simulink model "erg"  (R2021b)
settings: Solver=VariableStepAuto  StartTime=0.0  StopTime=TT  RelTol=1e-3
values from neighbouring files (symbols this model uses):
  A = [0,0,1,0 ... (first row only)    [erg_first_steps.m]
  B = [0,0 ... (first row only)    [erg_first_steps.m]
  constr = [10;10;0;0;0;0;0;0]    [erg_first_steps.m]
  delta = 1    [erg_first_steps.m]    (also in erg_point_testing.m = -1)
  Kd = 2*zeta*wn    [erg_first_steps.m]    (also in symplectic_euler.m = 2.556)
  Kp = umax/max(r)    [erg_first_steps.m]    (also in symplectic_euler.m = 3.3333)
  r = [11;9.9]    [erg_first_steps.m]    (also in erg_point_testing.m = [7;11])
  Ts = 0.1    [erg_first_steps.m]
  x0 = zeros(4,1)    [erg_first_steps.m]    (also in symplectic_euler.m = [0;0])
  zeta = 2    [erg_first_steps.m]    (also in erg_point_testing.m)
settings Model: Creator=jon-h  LastModifiedBy=jon-h

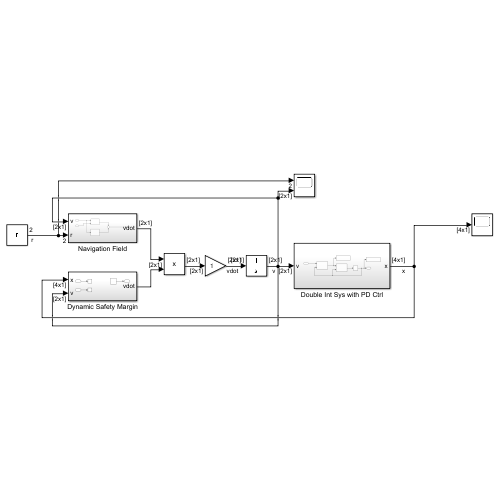
[thumbnail: Simulink's stored preview of the top-level diagram]
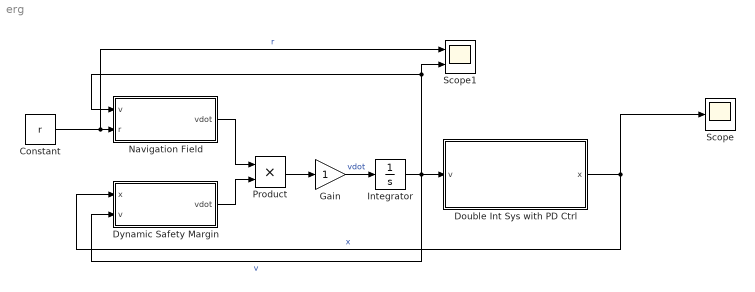
== system erg ==
  Constant : Constant  Value=r  SampleTime=Ts
  Double Int Sys with PD Ctrl : Subsystem
  Dynamic Safety Margin : Subsystem
  Gain : Gain
  Integrator : Integrator  InitialCondition=r
  Navigation Field : Subsystem
  Product : Product
  Scope : Scope
  Scope1 : Scope  NumInputPorts=2
  wires:
  Double Int Sys with PD Ctrl/1(x) -> Dynamic Safety Margin/1(x), Scope/1  "x"
  Integrator/1 -> Dynamic Safety Margin/2(v), Scope1/2, Navigation Field/1(v), Double Int Sys with PD Ctrl/1(v)  "v"
  Constant/1 -> Scope1/1, Navigation Field/2(r)  "r"
  Navigation Field/1(vdot) -> Product/1
  Dynamic Safety Margin/1(vdot) -> Product/2
  Gain/1 -> Integrator/1  "vdot"
  Product/1 -> Gain/1

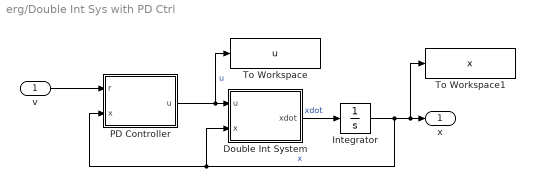
== system erg/Double Int Sys with PD Ctrl ==
  v : Inport
  Double Int System : MATLAB Function  TreatAsAtomicUnit=on
  Integrator : Integrator  InitialCondition=x0
  PD Controller : MATLAB Function  TreatAsAtomicUnit=on
  To Workspace : ToWorkspace  VariableName=u  SaveFormat=Timeseries  SampleTime=-1
  To Workspace1 : ToWorkspace  VariableName=x  SaveFormat=Timeseries  SampleTime=-1
  x : Outport
  wires:
  Integrator/1 -> To Workspace1/1, x/1, Double Int System/2(x), PD Controller/2(x)  "x"
  PD Controller/1(u) -> To Workspace/1, Double Int System/1(u)  "u"
  Double Int System/1(xdot) -> Integrator/1  "xdot"
  v/1 -> PD Controller/1(r)

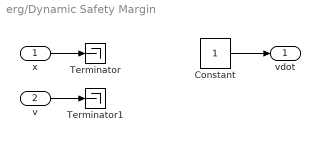
== system erg/Dynamic Safety Margin ==
  x : Inport
  v : Inport  Port=2
  Constant : Constant
  Terminator : Terminator
  Terminator1 : Terminator
  vdot : Outport
  wires:
  Constant/1 -> vdot/1
  x/1 -> Terminator/1
  v/1 -> Terminator1/1

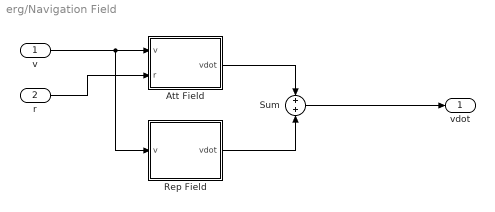
== system erg/Navigation Field ==
  v : Inport
  r : Inport  Port=2
  Att Field : MATLAB Function  TreatAsAtomicUnit=on
  Rep Field : MATLAB Function  TreatAsAtomicUnit=on
  Sum : Sum  Inputs=+|+
  vdot : Outport
  wires:
  v/1 -> Att Field/1(v), Rep Field/1(v)
  r/1 -> Att Field/2(r)
  Att Field/1(vdot) -> Sum/1
  Rep Field/1(vdot) -> Sum/2
  Sum/1 -> vdot/1

== matlab function erg/Double Int Sys with PD Ctrl/PD Controller ==
  data: r input; u output; x input; Kp parameter; Kd parameter
function u = fcn(r,x,Kp,Kd)

u = [ - Kp*(x(1)-r(1)) - Kd*x(3) ;
      - Kp*(x(2)-r(2)) - Kd*x(4) ];

== matlab function erg/Double Int Sys with PD Ctrl/Double Int System ==
  data: u input; xdot output; x input; A parameter; B parameter
function xdot = fcn(u,x,A, B)

xdot = A*x + B*u;

== matlab function erg/Navigation Field/Att Field ==
  data: v input; vdot output; r input; eta parameter
function vdot = fcn(v,r,eta)

vdot = (r-v) / max([norm(r-v), eta]);

== matlab function erg/Navigation Field/Rep Field ==
  data: v input; vdot output; constr parameter; delta parameter; zeta parameter
function vdot = fcn(v, constr, delta, zeta)

vdot = max( ( zeta - abs(v(1)-constr(1)) )/(zeta-delta) , 0.0 ) * (v(1)-constr(1))/norm(v(1)-constr(1)) + ...
       max( ( zeta - abs(v(2)-constr(2)) )/(zeta-delta) , 0.0 ) * (v(2)-constr(2))/norm(v(2)-constr(2));
